simulink model "RectifierBuckConverterTopology"  (R2021b)
settings: Solver=VariableStepAuto  StartTime=0.0  StopTime=5  MaxStep=1e-3  RelTol=1e-3
libraries: spsDiodeLib x7, spsMeanLib x4, spsACVoltageSourceLib x3, spsVoltageMeasurementLib x3, spsCurrentMeasurementLib x2, spsDCMachineLib x1, spsDCVoltageSourceLib x1, spsIGBTLib x1, slpidlib x1, eePowerMeasurement x1, spsSeriesRLCBranchLib x1, spsTriangleGeneratorLib x1
settings Model: Creator=pc3  LastModifiedBy=pc3
settings SolverCC: ZeroCrossAlgorithm=Adaptive
settings DebuggingCC: IgnoredZcDiagnostic=none

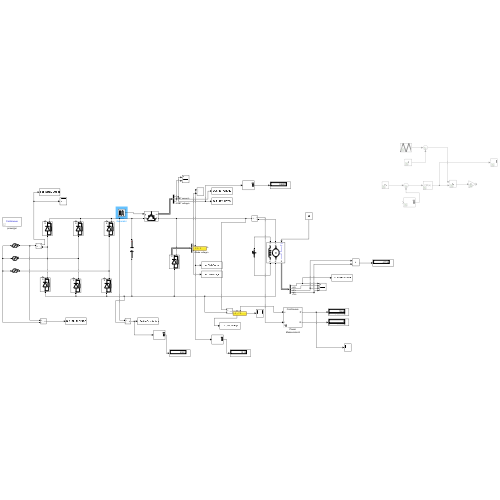
[thumbnail: Simulink's stored preview of the top-level diagram]
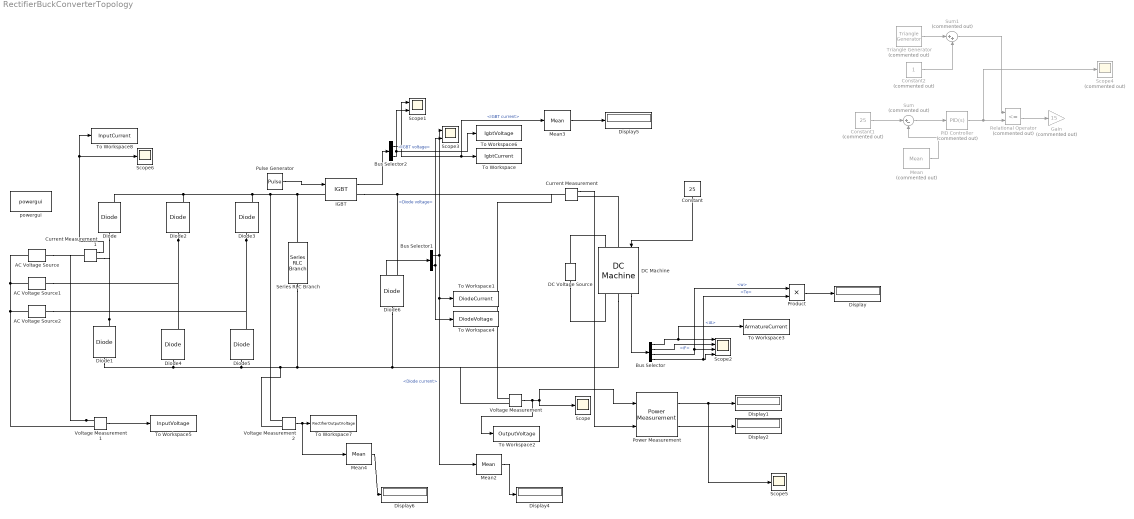
== system RectifierBuckConverterTopology ==
  AC Voltage Source : spsACVoltageSourceLib/AC Voltage Source  Amplitude=96*sqrt(2)  Phase=0  Frequency=50  SampleTime=0  Measurements=None  BusType=swing  Pref=10e3  Qref=0  Qmin=-inf  Qmax=+inf
  AC Voltage Source1 : spsACVoltageSourceLib/AC Voltage Source  Amplitude=96*sqrt(2)  Phase=120  Frequency=50  SampleTime=0  Measurements=None  BusType=swing  Pref=10e3  Qref=0  Qmin=-inf  Qmax=+inf
  AC Voltage Source2 : spsACVoltageSourceLib/AC Voltage Source  Amplitude=96*sqrt(2)  Phase=240  Frequency=50  SampleTime=0  Measurements=None  BusType=swing  Pref=10e3  Qref=0  Qmin=-inf  Qmax=+inf
  Bus Selector : BusSelector  OutputSignals=iA,iF,w,Te
  Bus Selector1 : BusSelector  OutputSignals=Diode current,Diode voltage
  Bus Selector2 : BusSelector  OutputSignals=IGBT current,IGBT voltage
  Constant : Constant  Value=25
  Constant1 : Constant  Commented=on  Value=25
  Constant2 : Constant  Commented=on
  Current Measurement : spsCurrentMeasurementLib/Current Measurement  PhasorSimulation=off  OutputType=Complex  PSBequivalent=0
  Current Measurement1 : spsCurrentMeasurementLib/Current Measurement  PhasorSimulation=off  OutputType=Complex  PSBequivalent=0
  DC Machine : spsDCMachineLib/DC Machine  PresetModel=No  MechanicalLoad=Torque TL  FieldType=Wound  ShowDetailedParameters=on  MeasurementBus=on  RLa="[ 0.8  0.0125]"  RLf="[ 210  23]"  Laf=1.8  MachineConstant=Torque constant (N.m/A)  Ke=1.8  Kt=1.8  J=1  Bm=0  Tf=0  w0=0  Ifinit=1.09523809518623  TsPowergui=0  TsBlock=-1
  DC Voltage Source : spsDCVoltageSourceLib/DC Voltage Source  Amplitude=230  Measurements=None
  Diode{,1..5} (6 alike) : spsDiodeLib/Diode  Ron=9.1e-3  Lon=0  Vf=1.04  IC=0  UseSnubber=0  Rs=500  Cs=250e-9  Measurements=on
  Diode6 : spsDiodeLib/Diode  Ron=19.6e-3  Lon=0  Vf=2.51  IC=0  UseSnubber=0  Rs=500  Cs=250e-9  Measurements=on
  Display{,1..2,4..6} (6 alike) : Display
  Gain : Gain  Commented=on  Gain=15
  IGBT : spsIGBTLib/IGBT  Ron=0.0588  Lon=0  Vf=1.6  Tf=1e-6  Tt=2e-6  IC=0  Rs=1e5  Cs=inf  Measurements=on
  Mean : spsMeanLib/Mean  Commented=on  Freq=5e3  Vinit=0  Ts=0
  Mean2 : spsMeanLib/Mean  Freq=60  Vinit=0  Ts=0
  Mean3 : spsMeanLib/Mean  Freq=5000  Vinit=0  Ts=0
  Mean4 : spsMeanLib/Mean  Freq=300  Vinit=0  Ts=0
  PID Controller : slpidlib/PID Controller  Commented=on  Controller=PID  Form=Parallel  TimeDomain=Continuous-time  UseExternalTs=off  SampleTime=-1  IntegratorMethod=Forward Euler  FilterMethod=Forward Euler  ControllerParametersSource=internal  P=1.7  I=0.5  D=0  UseFilter=on  N=100  TunerSelectOption=Transfer Function Based (PID Tuner App)  InitialConditionSource=internal  InitialConditionForIntegrator=0  InitialConditionForFilter=0  DifferentiatorICPrevScaledInput=0  ExternalReset=none  TrackingMode=off  Kt=1  LimitOutput=off  SatLimitsSource=internal  UpperSaturationLimit=inf  LowerSaturationLimit=-inf  LinearizeAsGain=on  AntiWindupMode=none  Kb=1  POutMin=[]  POutMax=[]  IOutMin=[]  IOutMax=[]  DOutMin=[]  DOutMax=[]  NOutMin=[]  NOutMax=[]  SumOutMin=[]  SumOutMax=[]  SaturationOutMin=[]  SaturationOutMax=[]  PParamMin=[]  PParamMax=[]  IParamMin=[]  IParamMax=[]  DParamMin=[]  DParamMax=[]  NParamMin=[]  NParamMax=[]  KbParamMin=[]  KbParamMax=[]  KtParamMin=[]  KtParamMax=[]  KbOutMin=[]  KbOutMax=[]  KtOutMin=[]  KtOutMax=[]  IntegratorOutMin=[]  IntegratorOutMax=[]  FilterOutMin=[]  FilterOutMax=[]  SumI1OutMin=[]  SumI1OutMax=[]  SumI2OutMin=[]  SumI2OutMax=[]  SumI3OutMin=[]  SumI3OutMax=[]  SumI4OutMin=[]  SumI4OutMax=[]  SumDOutMin=[]  SumDOutMax=[]  DifferentiatorOutMin=[]  DifferentiatorOutMax=[]  FilterDiffOutCoefMin=[]  FilterDiffOutCoefMax=[]  ReciprocalOutMin=[]  ReciprocalOutMax=[]  SumDenOutMin=[]  SumDenOutMax=[]  SumNumOutMin=[]  SumNumOutMax=[]  DivideOutMin=[]  DivideOutMax=[]  UdiffTsProdOutMin=[]  UdiffTsProdOutMax=[]  NTsProdOutMin=[]  NTsProdOutMax=[]  UintegralTsProdOutMin=[]  UintegralTsProdOutMax=[]  UngainTsProdOutMin=[]  UngainTsProdOutMax=[]  IntegratorContinuousStateAttributes=''  IntegratorStateMustResolveToSignalObject=off  IntegratorRTWStateStorageClass=Auto  FilterContinuousStateAttributes=''  FilterStateMustResolveToSignalObject=off  FilterRTWStateStorageClass=Auto  ParallelPVariant=InternalParameters  IdealPVariant=Disabled  IVariant=InternalParameters  DVariant=InternalParameters  IntegratorVariant=Continuous  SatVariant=Disabled  AWVariant=Passthrough  PCopyVariant=Disabled  TRVariant=Disabled  FdbkBlocksVariant=Forward  IdealPFdbkVariant=Disabled  SatFdbkVariant=Disabled  DerivativeFilterVariant=ContFilter  NVariant=InternalParameters  NCopyVariant=Disabled  FilterICVariant=InternalICsFilter  IntegratorICVariant=InternalICs  ExternalResetVariant=Disabled  TRSumVariant=Passthrough  SumFdbkVariant=Disabled  SumVariant=Sum_PID  TsampFilterVariant=InternalTs  TsampNgainVariant=Passthrough  TsampIntegralVariant=Passthrough  ExternalSaturationOutDataTypeStr=Inherit: Same as second input
  Power Measurement : eePowerMeasurement/Power Measurement  LabelModeActiveChoice=Continuous  F=50  K=[0 1 2 3]  Ts=0
      settings: SourceProductBaseCode=PS
  Product : Product
  Pulse Generator : DiscretePulseGenerator  PulseType=Time based  Amplitude=12  Period=1/5000  PulseWidth=20
  Relational Operator : RelationalOperator  Commented=on  Operator=<=  OutDataTypeStr=boolean  RndMeth=Simplest
  Scope : Scope
  Scope1 : Scope  NumInputPorts=2
  Scope2 : Scope  NumInputPorts=4
  Scope3 : Scope  NumInputPorts=2
  Scope4 : Scope  Commented=on
  Scope5 : Scope
  Scope6 : Scope
  Series RLC Branch : spsSeriesRLCBranchLib/Series RLC Branch  LConnTagsString=__new0  RConnTagsString=__new0  BranchType=C  Resistance=1  Inductance=1e-3  SetiL0=off  InitialCurrent=0  Capacitance=660e-6  Setx0=off  InitialVoltage=0  Measurements=None
  Sum : Sum  Commented=on  Inputs=|+-
  Sum1 : Sum  Commented=on  Inputs=|++
  To Workspace : ToWorkspace  VariableName=IgbtCurrent  SaveFormat=Timeseries  SampleTime=-1
  To Workspace1 : ToWorkspace  VariableName=DiodeCurrent  SaveFormat=Timeseries  SampleTime=-1
  To Workspace2 : ToWorkspace  VariableName=OutputVoltage  SaveFormat=Timeseries  SampleTime=-1
  To Workspace3 : ToWorkspace  VariableName=ArmatureCurrent  SaveFormat=Timeseries  SampleTime=-1
  To Workspace4 : ToWorkspace  VariableName=DiodeVoltage  SaveFormat=Timeseries  SampleTime=-1
  To Workspace5 : ToWorkspace  VariableName=InputVoltage  SaveFormat=Timeseries  SampleTime=-1
  To Workspace6 : ToWorkspace  VariableName=IgbtVoltage  SaveFormat=Timeseries  SampleTime=-1
  To Workspace7 : ToWorkspace  VariableName=RectifierOutputVoltage  SaveFormat=Timeseries  SampleTime=-1
  To Workspace8 : ToWorkspace  VariableName=InputCurrent  SaveFormat=Timeseries  SampleTime=-1
  Triangle Generator : spsTriangleGeneratorLib/Triangle Generator  Commented=on  Freq=5e3  Phase=0  Ts=0
  Voltage Measurement : spsVoltageMeasurementLib/Voltage Measurement  PhasorSimulation=off  OutputType=Complex  PSBequivalent=0
  Voltage Measurement1 : spsVoltageMeasurementLib/Voltage Measurement  PhasorSimulation=off  OutputType=Complex  PSBequivalent=0
  Voltage Measurement2 : spsVoltageMeasurementLib/Voltage Measurement  PhasorSimulation=off  OutputType=Complex  PSBequivalent=0
  powergui : spspowerguiLib/powergui  Priority=1  SimulationMode=Continuous  SampleTime=50e-6  frequency=60  Iterations=50  frequencyindice=50  Pbase=100e6  ErrMax=1e-4  UnitsV=kV  UnitsW=MW  buscounter=0  FunctionMessages=off  echomessages=off  EnableUseOfTLC=off  CurrentSourceSwitches=off  DisableSnubberDevices=off  DisableRonSwitches=off  DisableVfSwitches=off  DisplayEquations=off  AutomaticDiscreteSolvers=off  SolverType=Tustin/Backward Euler (TBE)  Interpol=off  ExternalGateDelay=off  methode=off  Ts=100  x0status=blocks  SPID=on  SwTol=0  HookPort=off  NonlinearTolerance=1e-4  nMaxIteration=100  ContinueOnMaxIteration=off  RestoreLinks=warning  ResistiveCurrentMeasurement=off  Frange=[0:2:500]  Ylog=off  Xlog=on  ShowGrid=off  save=off  variable=ZData  structure=0  ZoomFFT=off  StartTime=0.0  cycles=1  DisplayStyle=1  fundamental=60  FreqAxis=off  MaxFrequency=1000  frequencyindicesteady=1  RmsSteady=1  display=off
  wires:
  Mean4/1 -> Display6/1
  Bus Selector2/1 -> Scope1/1, Mean3/1, To Workspace/1  "<IGBT current>"
  Relational Operator/1 -> Gain/1
  Constant/1 -> DC Machine/1
  Constant1/1 -> Sum/1
  Voltage Measurement2/1 -> Mean4/1, To Workspace7/1
  Bus Selector1/2 -> Scope3/2, To Workspace4/1  "<Diode voltage>"
  Sum/1 -> PID Controller/1
  Voltage Measurement1/1 -> To Workspace5/1
  Bus Selector2/2 -> To Workspace6/1, Scope1/2  "<IGBT voltage>"
  Diode6/1 -> Bus Selector1/1
  Power Measurement/2 -> Display2/1
  Current Measurement1/1 -> Scope6/1, To Workspace8/1
  Product/1 -> Display/1
  DC Machine/1 -> Bus Selector/1
  PID Controller/1 -> Scope4/1, Relational Operator/2
  Mean/1 -> Sum/2
  Triangle Generator/1 -> Sum1/1
  Bus Selector1/1 -> Mean2/1, To Workspace1/1, Scope3/1  "<Diode current>"
  Mean2/1 -> Display4/1
  Bus Selector/3 -> Product/1, Scope2/3  "<w>"
  Bus Selector/2 -> Scope2/2  "<iF>"
  Bus Selector/4 -> Product/2, Scope2/4  "<Te>"
  Constant2/1 -> Sum1/2
  Bus Selector/1 -> To Workspace3/1, Scope2/1  "<iA>"
  Pulse Generator/1 -> IGBT/1
  Current Measurement/1 -> Power Measurement/2
  Power Measurement/1 -> Scope5/1, Display1/1
  IGBT/1 -> Bus Selector2/1
  Sum1/1 -> Relational Operator/1
  Mean3/1 -> Display5/1
  Voltage Measurement/1 -> To Workspace2/1, Scope/1, Power Measurement/1
  connections:
  Diode6/LConn1 -- Voltage Measurement/LConn2 -- DC Machine/RConn1 -- Series RLC Branch/RConn1 -- Voltage Measurement2/LConn2 -- Diode5/LConn1 -- Diode1/LConn1 -- Diode4/LConn1
  IGBT/RConn1 -- Diode6/RConn1 -- Current Measurement/LConn1 -- Voltage Measurement/LConn1
  IGBT/LConn1 -- Diode/RConn1 -- Diode2/RConn1 -- Diode3/RConn1 -- Voltage Measurement2/LConn1 -- Series RLC Branch/LConn1
  Diode3/LConn1 -- Diode5/RConn1 -- AC Voltage Source2/RConn1
  AC Voltage Source/LConn1 -- Voltage Measurement1/LConn2 -- AC Voltage Source2/LConn1 -- AC Voltage Source1/LConn1
  Diode2/LConn1 -- Diode4/RConn1 -- AC Voltage Source1/RConn1
  Diode1/RConn1 -- Diode/LConn1 -- Current Measurement1/RConn1
  Voltage Measurement1/LConn1 -- AC Voltage Source/RConn1 -- Current Measurement1/LConn1
  DC Machine/LConn1 -- Current Measurement/RConn1
  DC Voltage Source/LConn1 -- DC Machine/RConn2
  DC Voltage Source/RConn1 -- DC Machine/LConn2
